simulink model "bubblechase"  (R2015a)
settings: Solver=ode4  SolverMode=MultiTasking  StartTime=0.0  StopTime=inf  FixedStep=BKIN_STEP_TIME  RelTol=1e-3
StartFcn:
  |  warndlg('Dexterit-E models cannot run under simulation. Please compile your model and run it from within Dexterit-E.');set_param(bdroot,'SimulationCommand','stop')
model workspace (MAT data in the model file):
  BKIN_STEP_TIME = 0.00025
  col_x = 1
  col_y = 2
  E_TARGET_ON = 3
  LOGICAL_RADIUS = 4
  START_TARGET_COL = 1
  END_TARGET_COL = 2
  DELAY_POSTTRIAL_COL = 6
  E_STAY_CENTER = 2
  VISUAL_RADIUS = 3
  COLOR = 5
  K_SCORETEXT_ROW = 1
  LABEL_HEIGHT = 9
  E_HIT_TARGET = 5
  E_MISS_TARGET = 9
  K_REWARD_VAL = 2
  K_VIS_RAD = 3
  E_REWARD = 6
  WAIT_AT_START_COL = 3
  LABEL = 8
  K_SCORE_TIME = 4
  HAND_VIS_COL = 9
  DO_REWARD_COL = 10
  E_SHOW_SCORE = 17
  DISPLAY_TRIAL_COL = 11
  BKIN_KINEMATIC_FRAME_SIZE = 400
  E_NO_EVENT = 0
  PAUSE_TIME_COL = 4
  MAXREACH_TIME_COL = 5
  TARGET_XVEL_COL = 7
  TARGET_YVEL_COL = 8
  K_POP_TIME = 5
  K_POP_R_EXPAND = 6
  K_POP_FADE = 7
  STROKE_WIDTH = 6
  STROKE_COLOR = 7
  K_MAX_DIST = 8
  E_TARGET_ESCAPE = 11
  E_END_BREAK = 20
  BTN_BREAK = 2
undefined symbols (not defined in the file or in its folder): slselsubs
libraries: Video x4, General x3, slrtlib x3, simulink x2, KINARM_general x1, xpcnilib x1
(part 1 of 2)
CloseFcn:
  | rtwprivate ssgencode ModelCloseRequest b2lab2d
settings Model: ModifiedComment=chris -- Wed Feb 16 09:18:30 2005 -- Version 1.1384  ModifiedHistory=Feb 16/05 - Add error repeat, add offset ramp  ExtModeArmWhenConnect=off  ExtModeLogAll=off  Creator=Chris Grebeldinger  LastModifiedBy=User
settings SolverCC: EnableConcurrentExecution=on  AutoInsertRateTranBlk=on
settings DataIOCC: LimitDataPoints=off  SignalLoggingSaveFormat=ModelDataLogs  SaveOutput=off  SaveTime=off  SignalLoggingName=sigsOut
settings OptimizationCC: BlockReduction=off  BooleanDataType=off  OptimizeBlockIOStorage=off  BufferReuse=off  GlobalBufferReuse=off  ExpressionFolding=off  ExpressionDepthLimit=2147483647  LocalBlockOutputs=off  InitFltsAndDblsToZero=on
settings DebuggingCC: SaveWithParameterizedLinksMsg=none  UnderspecifiedInitializationDetection=Classic  MergeDetectMultiDrivingBlocksExec=none  SignalResolutionControl=TryResolveAllWithWarning  MultiTaskDSMMsg=warning  FcnCallInpInsideContextMsg=UseLocalSettings  StateNameClashWarn=warning  StrictBusMsg=ErrorOnBusTreatedAsVector
settings HardwareCC: ProdIntDivRoundTo=Zero  ProdEndianess=LittleEndian  ProdLongLongMode=on  ProdHWDeviceType=Generic->32-bit x86 compatible  TargetHWDeviceType=32-bit Generic
settings SFSimCC: SimParseCustomCode=off
settings RTWCC: SystemTargetFile=slrt.tlc  TemplateMakefile=slrt_default_tmf  Description=Simulink Real-Time  CustomSourceCode="#include \"stdio.h\""  RTWCompilerOptimization=on
settings CodeAppCC: MaxIdLength=63
settings SimulinkRealTimeCC: TargetFcnLib=ansi_tfl_tmw.mat  GeneratePreprocessorConditionals=Disable all  xPCisDownloadable=off

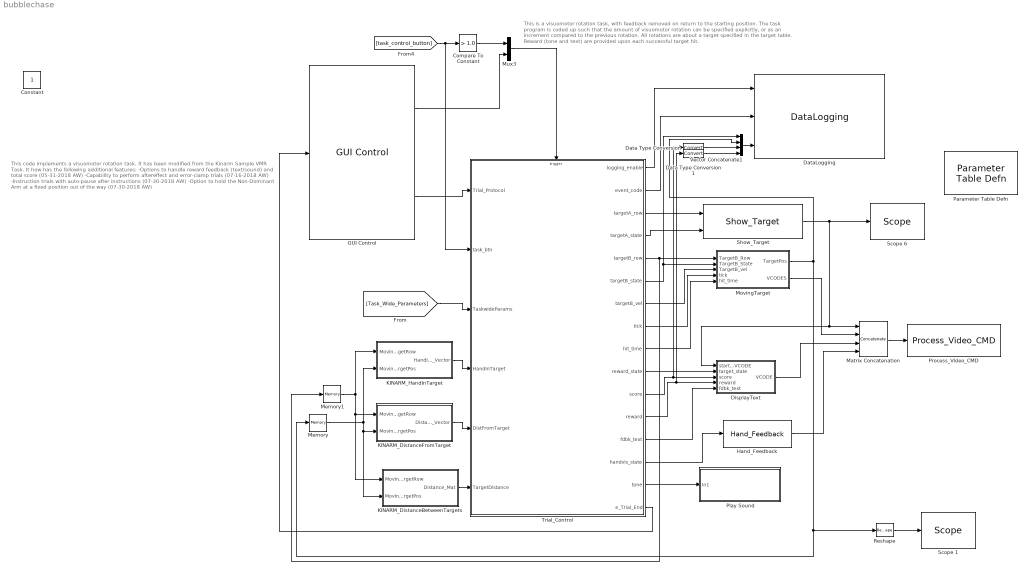
== system bubblechase ==
  note: This code implements a visuomotor rotation task. It has been modified from the Kinarm Sample VMR Task. It how has the following additional features:
      |
      | -Options to handle reward feedback (text/sound) and total score (05-31-2018 AW)
      | -Capability to perform aftereffect and error-clamp trials (07-16-2018 AW)
      | -Instruction trials with auto-pause after instructions (07-30-2018 AW)
      | -Option to hold the Non-Dominant Arm at a fixed position out of the way (07-30-2018 AW)
  note: This is a visuomotor rotation task, with feedback removed on return to the starting position.
      | The task program is coded up such that the amount of visuomotor rotation can be specified explicitly, or as an increment compared to the previous rotation.
      | All rotations are about a target specified in the target table.
      |
      | Reward (tone and text) are provided upon each successful target hit.
  Compare To Constant : simulink/Logic and Bit Operations/Compare To Constant  relop=>  const=1.0  OutDataTypeStr=boolean
  Data Type Conversion : DataTypeConversion
  Data Type Conversion1 : DataTypeConversion
  DataLogging : General/DataLogging  log_event_codes=on  log_analog_inputs=on  show_time_remaining=off  ecat_include=on
  DisplayText : Subsystem
  GUI Control : General/GUI Control  task_version=1.0  show_repeat_trial_flag=off  use_custom_tp=off  target_type_str=Circle  Target_Type=1  XYcols=[1 2]  Vcols=3  Lcols=4  indices_padding=[0 0 0 0;0 0 0 0]  target_table_rows=32  load_table_rows=20  tp_table_rows=50
  Hand_Feedback : KINARM_general/Hand_Feedback  feedback_cntl_src=status only
  KINARM_DistanceBetweenTargets : Subsystem
  KINARM_DistanceFromTarget : Subsystem  mask(KINARM_DistanceFromTarget){use_dominant_hand=on}
      mask prompts: use_dominant_hand "Use "arm to be assessed"?"
      mask help: This block returns a vector corresponding to the Target_Table rows indicating the distance from the specified hand to the center of each of the targets.
      mask init:
      | block_path = gcb;  % store block path, as gcb may change with block operations
      | 
      | %%% Handle background colours if link status changes.  
      | checkBackgroundColour(block_path, 'KINARM_general');
      mask Help:
      | Used to determine the distance from hand (fingertip) to center of targets in the Target_Table.
      | <P>
      | <H2>Library </H2>
      | KINARM general
      | 
      | <H2>Description </H2>
      | This block returns a vector corresponding to the Target_Table rows indicating the distance from the specified hand (fingertip) to the center of each of the targets.
      | <P>
      | The output vector is typically used by a Stateflow chart to affect behavior of the system.  Because this block returns distance-from-target information for all targets in the Target Table, multiple targets can be monitored at once (i.e. the Stateflow chart could have certain transitions that occur if the hand is a given distance from one target versus the distance from a separate target).
      | <P>
      | Because the KINARM_DistanceFromTarget block returns information for only one hand, two copies of this block are required if information for both hands is desired.
      | 
      | <H2>Parameters and Dialog Box</H2>
      | <B>Use "arm to be assessed"?:</B> this checkbox determines which hand is used by this block. In Dexterit-E the operator selects the "arm to be assessed" using radio buttons.
      | When this box is checked the output of this block is derived from the hand information corresponding to the arm selection made by the operator in Dexterit-E.
      | When this box is unchecked the output of this block is derived from the contralateral arm.
      | (Note: to obtain information about both hands, then 2 separate copies of this block are required - one for each hand.)
      | <H2>Related Blocks </H2>
      | DataLogging<BR>
      | KINARM_HandInTarget
  KINARM_HandInTarget : Subsystem  mask(KINARM_HandInTarget){use_dominant_hand=on, target_type=Circle, num_states=1, attribcol1=[LOGICAL_RADIUS], attribcol2=[3], attribcol3=[3], attribcol4=[3], attribcol5=[0]}
      mask prompts: use_dominant_hand "Use "arm to be assessed"?"; target_type "Type of Target"; num_states "Number of Target States"; attribcol1 "State 1 Target Table Column(s)"; attribcol2 "State 2 Target Table Column(s)"; attribcol3 "State 3 Target Table Column(s)"; attribcol4 "State 4 Target Table Column(s)"; attribcol5 "State 5 Target Table Column(s)"
      mask help: This block returns a vector or array corresponding to the Target_Table rows indicating whether the specified hand is in (=1) or out (=0) of each of the targets.
      mask init:
      | block_path = gcb;  % store block path, as gcb may change with block operations
      | 
      | %%% Get the model's workspace, because it is required to evaluate constants from the Parameter Table Def'n block
      | modelName=bdroot(block_path);
      | modelWorkspace = get_param(modelName, 'ModelWorkspace');
      | 
      | %%% Handle background colours if link status changes.  
      | checkBackgroundColour(block_path, 'KINARM_general');
      | 
      | %%% create the names of the input and output ports to display on the mask
      | % Select only the desired states for output. The output port is also renamed to reflect 
      | % whether the output is a vector (in the case of a single state) or an array (of vectors, 
      | % one for each of multiple states).
      | 
      | numStates = str2double( get_param(block_path, 'num_states') );
      | 
      | if numStates == 1
      | 	set_param([block_path '/Selected States'], 'Value', '[1]');
      | 	outputname = 'HandInTarget_Vector';
      | elseif numStates == 2
      | 	set_param([block_path '/Selected States'], 'Value', '[1,2]');
      | 	outputname = 'HandInTarget_Array';
      | elseif numStates == 3
      | 	set_param([block_path '/Selected States'], 'Value', '[1,2,3]');
      | 	outputname = 'HandInTarget_Array';
      | elseif numStates == 4
      | 	set_param([block_path '/Selected States'], 'Value', '[1,2,3,4]');
      | 	outputname = 'HandInTarget_Array';
      | else
      | 	set_param([block_path '/Selected States'], 'Value', '[1,2,3,4,5]');
      | 	outputname = 'HandInTarget_Array';
      | end
      | output_block=char(find_system(gcb,'LookUnderMasks','all','FollowLinks','on','SearchDepth',1,'BlockType','Outport'));
      | set_param(output_block, 'Name', outputname);
      | 
      | 
      | %%%%%%%%%%%%%%%%%%%%%%%%%%%%%%%%%%%%%%%%%%%%%%%%%%%%%%%%%%%%%
      | %%% Check and format the input strings for the vectors of column entires
      | targetTypeStr=get_param(block_path, 'target_type');
      | 
      | switch targetTypeStr(1:3)
      | 	case 'Cir',		numCol = 1;
      | 	case 'Ell',		numCol = 3;
      |     case 'Rec',		numCol = 3;
      |     case 'Lin',		numCol = 3;
      |     case 'Tri',		numCol = 4;
      | 	otherwise,		numCol = 1;
      | end
      | 
      | for ii = 1:5
      | 	variableName = ['attribcol' num2str(ii)];
      | 	attribcoltext = get_param(block_path, variableName);
      | 	attribcoltext = checkUserInputVectorLength(attribcoltext, numCol);
      | 	set_param(block_path, variableName, attribcoltext);
      | end
      | 
      | 
      | %%%%%%%%%%%%%%%%%%%%%%%%%%%%%%%%%%%%%%%%%%%%%%%%%%%%%%%%%%%%%
      | %%% Create the text to show on the mask
      | numStates = str2num(get_param(block_path, 'num_states'));
      | columntext='(columns: ';
      | 
      | for ii = 1:numStates
      | 	variableName = ['attribcol' num2str(ii)];
      | 	attribcolString = get_param(block_path, variableName);
      | 	if isempty(modelWorkspace)
      | 		% if the block is part of a library, then modelWorkspace will be empty and the other code to evaluate attribcolStringEval will fail
      | 		attribcolStringEval = '3';
      | 	else
      | 		[attribcolValue, errorMessage] = BKINevalin(modelWorkspace, attribcolString);
      | 		attribcolStringEval = mat2str( attribcolValue );
      | 	end
      | 	if ii > 1
      | 		columntext = [columntext, '; ', attribcolStringEval];
      | 	else
      | 		columntext = [columntext, attribcolStringEval];
      | 	end
      | end
      | 
      | % Add formatting spaces so that the mask looks nice
      | columntext=strvcat([columntext ')'],' ', ' ');
      mask Help:
      | Used to determine if the hand (fingertip) is in any of the targets in the Target_Table.
      | <P>
      | <B><I>Use of this block requires that the DataLogging block (General library) be set to log KINARM data.</I></B>
      | 
      | <H2>Library </H2>
      | KINARM general
      | 
      | <H2>Description </H2>
      | This block returns a vector or array corresponding to the Target_Table rows indicating whether the specified hand (i.e. fingertip) is in or out of each of the targets.  Each element in the output vector or output array will be either a 0 (hand not in target) or a 1 (hand in target).
      | <P>
      | A vector is returned if only one target state is specified in each target row (see Parameters and Dialog Box), with each index of the vector corresponding to a row in the target table.  An array is returned if more than one target state is specified in a target row, with each row of the array corresponding to a target row and each column corresponding to the nth target state specified in each target row.
      | <P>
      | The output vector or array is typically used by a stateflow chart to affect behavior of the system.  Because this block returns hand-in-target information for all targets in the target table, multiple targets can be monitored at once (i.e. the Stateflow chart could have certain transitions that occur if the hand is in one target and other transitions if it is in a different target).  Likewise, because this block returns hand-in-target information for multiple states of a single target, those multiple states can be monitored simultaneously.
      | <P>
      | Because the KINARM_HandInTarget block returns information for only one hand, two copies of this block are required if information for both hands is desired.
      | <P>
      | 
      | <H2>Parameters and Dialog Box</H2>
      | <B>Use "arm to be assessed"?:</B> this checkbox determines which hand is used by this block. In Dexterit-E the operator selects the "arm to be assessed" using radio buttons.
      | When this box is checked the output of this block is derived from the hand information corresponding to the arm selection made by the operator in Dexterit-E.
      | When this box is unchecked the output of this block is derived from the contralateral arm.
      | (Note: to obtain information about both hands, then 2 separate copies of this block are required - one for each hand.)
      | <P>
      | <B>Type of Target:</B> Enter the type of target specified in the target table:
      | <P>
      | <B>Number of Target States:</B> Enter the number of target states specified in each target row.  Up to four target states are allowed per target row.
      | <P>
      | <B>State <n> Target Table Columns:</B> Enter the columns in the Target Table that specify the relevant target attributes.  Do this for each target state.
      | For a circle, enter the columns corresponding to logical radius (e.g. 4)
      | <BR>For an ellipse, enter the columns corresponding to major radius, minor radius, rotation angle (e.g. [4, 5, 6]).
      | <BR>For a rectangle, enter the columns corresponding to length, height, and rotation angle (e.g. [4, 5, 6]).
      | <BR>For a line, enter the columns corresponding to stroke width, endpoint in x, and endpoint in y (e.g. [3, 4, 5]).
      | <BR>For a triangle, enter the columns corresponding to length, height, peak offset, and rotation angle (e.g. [4, 5, 6, 7]).
      | 
      | <H2>Examples</H2>
      | <B>Example 1.</B>  Suppose a target row will be used to define 1 state for a circle type target and the radius of the visual target is the same radius to be used for determination of hand-in-target.  The related Target Table column is: column 6 = radius.  For this example, "State 1 Target Table Columns" would equal [6].
      | <P>
      | 
      | <B>Example 2.</B>  Suppose a target row will be used to define 1 state for a circle type target, but the radius of the visual target will be different than the radius to be used for determination of hand-in-target.  This option allows independent control over the size of the visual target versus the accuracy needed to be considered "in the target".  The related Target Table columns are: column 6 = radius1 (i.e. radius to target to be drawn); column 7 = radius2 (i.e. radius to be used for hand-in-target) .  For this example, "State 1 Target Table Columns" would equal [7].
      | <P>
      | <B>Example 3.</B>  Suppose a target row will be used to define 2 states for a circle type target, where the radius of the visual target will be a constant, but depending on the state of the system, one of 2 other and different radii will be used for determination of hand-in-target.  The related Target Table columns are: column 6 = radius1 (i.e. radius to target to be drawn); column 7 = radius2 (i.e. radius to be used for hand-in-target for state 1); column 8 = radius3 (i.e. radius to be used for hand-in-target for state 2).  For this example, "State 1 Target Table Columns" would equal [7], while "State 2 Target Table Columns" would equal [8].
      | <P>
      | 
      | <H2>Related Blocks </H2>
      | DataLogging
      mask TypeOptions target_type: Circle | Ellipse | Rectangle | Line | Triangle
      mask Callback target_type:
      | %%%%
      | % Because of bugs iN R2007, R2010a and R2013a (which have been reported to Mathworks), the following code
      | % is required here because in the Initialization Section it will ONLY correctly update those Mask Parameters that are hidden
      | % when the OK button is clicked (NOTE: the initialization code will correctly update all Mask Parameters when the Apply button
      | % is clicked, the bug is that it should also update everything when the OK button is clicked in the absence of an Apply click)
      | %
      | % Adding a set_param call which updates one of the mask parameters will call the initialization code to run, which "avoids"
      | % this bug. This code should be removed once Mathworks has fixed this bug.
      | 
      | temp = get_param(gcb, 'target_type');
      | set_param(gcb, 'target_type', temp);
      mask TypeOptions num_states: 1 | 2 | 3 | 4 | 5
      mask Callback num_states:
      | num_states = str2num(get_param(gcb, 'num_states'));
      | vis = get_param(gcb, 'MaskVisibilities');
      | 
      | % Select only the desired states for output. The output port is also renamed to reflect
      | % whether the output is a vector (in the case of a single state) or an array (of vectors,
      | % one for each of multiple states).
      | output_block=char(find_system(gcb, 'LookUnderMasks', 'all', 'FollowLinks', 'on', 'SearchDepth', 1, 'BlockType', 'Outport'));
      | 
      | if num_states == 1
      | % % % 	set_param([gcb '/Selected States'], 'Value', '[1]');
      | % % % 	set_param(output_block, 'Name', 'HandInTarget_Vector');
      | 	vis{5} = 'off';
      | 	vis{6} = 'off';
      | 	vis{7} = 'off';
      | 	vis{8} = 'off';
      | elseif num_states == 2
      | % % % 	set_param([gcb '/Selected States'], 'Value', '[1,2]');
      | % % % 	set_param(output_block, 'Name', 'HandInTarget_Array');
      | 	vis{5} = 'on';
      | 	vis{6} = 'off';
      | 	vis{7} = 'off';
      | 	vis{8} = 'off';
      | elseif num_states == 3
      | % % % 	set_param([gcb '/Selected States'], 'Value', '[1,2,3]');
      | % % % 	set_param(output_block, 'Name','HandInTarget_Array');
      | 	vis{5} = 'on';
      | 	vis{6} = 'on';
      | 	vis{7} = 'off';
      | 	vis{8} = 'off';
      | elseif num_states == 4
      | % % % 	set_param([gcb '/Selected States'], 'Value', '[1,2,3,4]');
      | % % % 	set_param(output_block, 'Name','HandInTarget_Array');
      | 	vis{5} = 'on';
      | 	vis{6} = 'on';
      | 	vis{7} = 'on';
      | 	vis{8} = 'off';
      | else
      | % % % 	set_param([gcb '/Selected States'], 'Value', '[1,2,3,4,5]');
      | % % % 	set_param(output_block, 'Name', 'HandInTarget_Array');
      | 	vis{5} = 'on';
      | 	vis{6} = 'on';
      | 	vis{7} = 'on';
      | 	vis{8} = 'on';
      | end
      | set_param(gcb, 'MaskVisibilities', vis);
      mask Display:
      | disp(columntext);
      | port_label('output',1,outputname);
  Matrix Concatenation : Concatenate  NumInputs=4  Mode=Multidimensional array
  Memory : Memory  InheritSampleTime=on
  Memory1 : Memory  InheritSampleTime=on
  MovingTarget : Subsystem
  Mux3 : Mux  Inputs=2
  Parameter Table Defn : General/Parameter Table Defn  ShowInLibBrowser=0
  Play Sound : Subsystem
  Process_Video_CMD : Video/Process_Video_CMD  video_delay=50
  Reshape : Reshape
  Scope 1 : slrtlib/Displays and Logging/Scope   scopeno=6  scopetype=Target  autostart=on  viewmode=Numerical  formatstr='%15.6f'  grid=on  ylimits=[0,0]  nosamples=250  noprepostsamples=0  interleave=1  triggermode=FreeRun  triggersignal=1  trigsignalfromport=off  triggerlevel=0.0  triggerslope=Either  triggerscope=1  triggersample=0  filename=data.dat  mode=Lazy  writesize=512  autorestart=off  dynamicfilemode=off  maxwritefilesize=512*1024^2
  Scope 6 : slrtlib/Displays and Logging/Scope   scopeno=4  scopetype=Target  autostart=on  viewmode=Numerical  formatstr='%15.6f'  grid=on  ylimits=[0,0]  nosamples=250  noprepostsamples=0  interleave=1  triggermode=FreeRun  triggersignal=1  trigsignalfromport=off  triggerlevel=0.0  triggerslope=Either  triggerscope=1  triggersample=0  filename=data.dat  mode=Lazy  writesize=512  autorestart=off  dynamicfilemode=off  maxwritefilesize=512*1024^2
  Show_Target : Video/Show_Target  target_type=Circle  num_states=1  attribcol1=[COLOR 0 0 VISUAL_RADIUS]  attribcol2=[0 0 0 0]  attribcol3=[0 0 0 0]  attribcol4=[0 0 0 0]  attribcol5=[0 0 0 0]  stateindices_padding=[0 0 0 0 0 0 0;0 0 0 0 0 0 0;0 0 0 0 0 0 0;0 0 0 0 0 0 0;0 0 0 0 0 0 0]  source=dialog  opacity=100  target_display=Both subject and operator displays  num_col=4
  Trial_Control : Stateflow chart  TreatAsAtomicUnit=on
  Vector Concatenate1 : Concatenate  NumInputs=4
  Constant : Constant  IOType=siggen
  wires:
  Show_Target/1 -> Scope 6/1, DisplayText/1(start_tgt_VCODE), Matrix Concatenation/1
  GUI Control/2 -> Trial_Control/1(Trial_Protocol)
  Trial_Control/16(e_Trial_End) -> GUI Control/1
  Trial_Control/4(targetA_state) -> Show_Target/2
  Trial_Control/3(targetA_row) -> Show_Target/1
  Trial_Control/6(targetB_state) -> MovingTarget/2(TargetB_State), Vector Concatenate1/1
  Trial_Control/2(event_code) -> DataLogging/2
  Matrix Concatenation/1 -> Process_Video_CMD/1
  Hand_Feedback/1 -> Matrix Concatenation/4
  MovingTarget/1(TargetPos) -> Memory/1, Reshape/1, Vector Concatenate1/2
  Trial_Control/1(logging_enable) -> DataLogging/1
  Trial_Control/10(reward_state) -> DisplayText/2(target_state)
  Trial_Control/11(score) -> DisplayText/3(score), Data Type Conversion/1
  [Task_Wide_Parameters] -> Trial_Control/3(TaskwideParams)
  Trial_Control/12(reward) -> Data Type Conversion1/1, DisplayText/4(reward)
  Reshape/1 -> Scope 1/1
  Memory/1 -> KINARM_DistanceFromTarget/2(MovingTargetPos), KINARM_DistanceBetweenTargets/2(MovingTargetPos), KINARM_HandInTarget/2(MovingTargetPos)
  Trial_Control/13(fdbk_text) -> DisplayText/5(fdbk_text)
  DisplayText/1(VCODE) -> Matrix Concatenation/3
  GUI Control/1 -> Mux3/2
  Vector Concatenate1/1 -> DataLogging/3
  Trial_Control/5(targetB_row) -> Memory1/1, MovingTarget/1(TargetB_Row)
  Trial_Control/7(targetB_vel) -> MovingTarget/3(TargetB_vel)
  Trial_Control/8(tick) -> MovingTarget/4(tick)
  MovingTarget/2(VCODES) -> Matrix Concatenation/2
  Trial_Control/14(handvis_state) -> Hand_Feedback/1
  KINARM_HandInTarget/1(HandInTarget_Vector) -> Trial_Control/4(HandInTarget)
  Memory1/1 -> KINARM_HandInTarget/1(MovingTargetRow), KINARM_DistanceBetweenTargets/1(MovingTargetRow), KINARM_DistanceFromTarget/1(MovingTargetRow)
  KINARM_DistanceFromTarget/1(Distance_Vector) -> Trial_Control/5(DistFromTarget)
  KINARM_DistanceBetweenTargets/1(Distance_Mat) -> Trial_Control/6(TargetDistance)
  Trial_Control/9(hit_time) -> MovingTarget/5(hit_time)
  Trial_Control/15(tone) -> Play Sound/1(In1)
  Data Type Conversion/1 -> Vector Concatenate1/3
  Data Type Conversion1/1 -> Vector Concatenate1/4
  [task_control_button] -> Trial_Control/2(task_btn), Compare To Constant/1
  Mux3/1 -> Trial_Control/Trigger
  Compare To Constant/1 -> Mux3/1

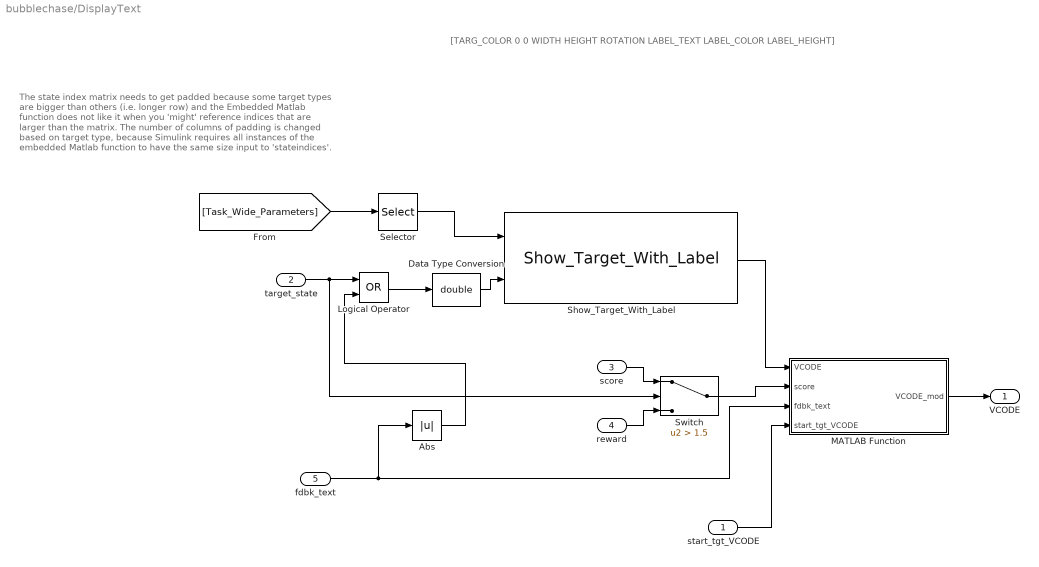
== system bubblechase/DisplayText ==
  note: [TARG_COLOR 0 0 WIDTH HEIGHT ROTATION LABEL_TEXT LABEL_COLOR LABEL_HEIGHT]
  note: The state index matrix needs to get padded because
      | some target types are bigger than others (i.e. longer row)
      | and the Embedded Matlab function does not like it when you
      |  'might' reference indices that are larger than the matrix.
      |
      | The number of columns of padding is changed based on target
      | type, because Simulink requires all instances of the embedded
      | Matlab function to have the same size input to 'stateindices'.
  start_tgt_VCODE : Inport  OutDataTypeStr=double
  target_state : Inport  Port=2  OutDataTypeStr=double
  score : Inport  Port=3  OutDataTypeStr=int32
  reward : Inport  Port=4  OutDataTypeStr=int32
  fdbk_text : Inport  Port=5  OutDataTypeStr=int32
  Abs : Abs
  Data Type Conversion : DataTypeConversion  OutDataTypeStr=double
  Logical Operator : Logic  Operator=OR  AllPortsSameDT=off  OutDataTypeStr=boolean
  MATLAB Function : MATLAB Function  TreatAsAtomicUnit=on
  Selector : Selector  Indices=[K_SCORETEXT_ROW]
  Show_Target_With_Label : Video/Show_Target_With_Label  target_type=Rectangle  num_states=1  attribcol1=[COLOR 0 0 VISUAL_RADIUS VISUAL_RADIUS 0 LABEL COLOR LABEL_HEIGHT]  attribcol2=[0 0 0 0 0 0 0 0 0]  attribcol3=[0 0 0 0 0 0 0 0 0]  attribcol4=[0 0 0 0 0 0 0 0 0]  attribcol5=[0 0 0 0 0 0 0 0 0]  stateindices_padding=[0 0;0 0;0 0;0 0;0 0]  source=dialog  opacity=100  target_display=Both subject and operator displays
  Switch : Switch  Criteria=u2 > Threshold  Threshold=1.5
  VCODE : Outport
  wires:
  target_state/1 -> Logical Operator/1, Switch/2
  Show_Target_With_Label/1 -> MATLAB Function/1(VCODE)
  MATLAB Function/1(VCODE_mod) -> VCODE/1
  score/1 -> Switch/1
  reward/1 -> Switch/3
  Switch/1 -> MATLAB Function/2(score)
  [Task_Wide_Parameters] -> Selector/1
  Selector/1 -> Show_Target_With_Label/1
  fdbk_text/1 -> Abs/1, MATLAB Function/3(fdbk_text)
  Abs/1 -> Logical Operator/2
  Logical Operator/1 -> Data Type Conversion/1
  Data Type Conversion/1 -> Show_Target_With_Label/2
  start_tgt_VCODE/1 -> MATLAB Function/4(start_tgt_VCODE)

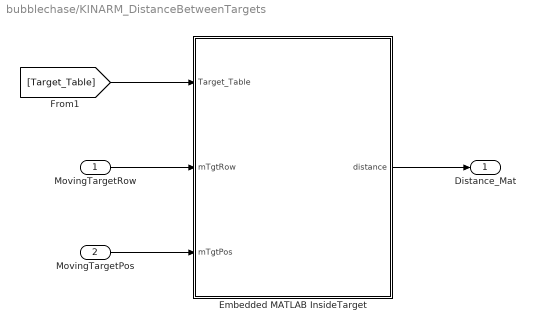
== system bubblechase/KINARM_DistanceBetweenTargets ==
  MovingTargetRow : Inport
  MovingTargetPos : Inport  Port=2
  Embedded MATLAB InsideTarget : MATLAB Function  TreatAsAtomicUnit=on
  Distance_Mat : Outport
  wires:
  Embedded MATLAB InsideTarget/1(distance) -> Distance_Mat/1
  [Target_Table] -> Embedded MATLAB InsideTarget/1(Target_Table)
  MovingTargetRow/1 -> Embedded MATLAB InsideTarget/2(mTgtRow)
  MovingTargetPos/1 -> Embedded MATLAB InsideTarget/3(mTgtPos)

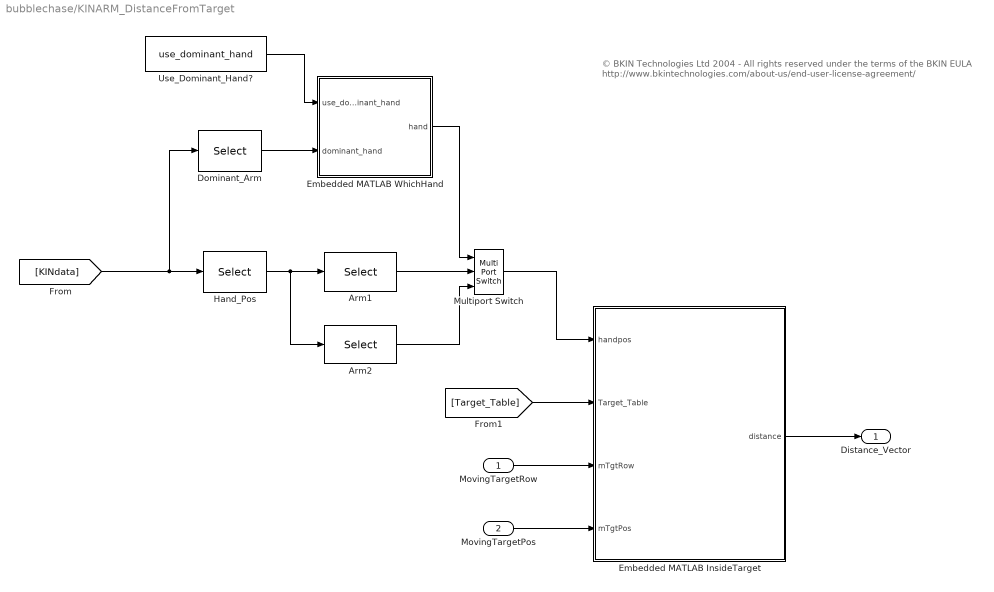
== system bubblechase/KINARM_DistanceFromTarget ==
  note: © BKIN Technologies Ltd 2004  - All rights reserved under the terms of the BKIN EULA
      | http://www.bkintechnologies.com/about-us/end-user-license-agreement/
  MovingTargetRow : Inport
  MovingTargetPos : Inport  Port=2
  Arm1 : Selector  NumberOfDimensions=2  InputPortWidth=3  IndexOptions=Index vector (dialog),Select all  Indices=1,-1  OutputSizes=slselsubs([(-2),(-2)],1),slselsubs([(-2),(-2)],2)
  Arm2 : Selector  NumberOfDimensions=2  InputPortWidth=3  IndexOptions=Index vector (dialog),Select all  Indices=2,-1  OutputSizes=slselsubs([(-2),(-2)],1),slselsubs([(-2),(-2)],2)
  Dominant_Arm : Selector  NumberOfDimensions=2  InputPortWidth=3  IndexOptions=Index vector (dialog),Index vector (dialog)  Indices=[3],[1]  OutputSizes=slselsubs([(-2),(-2)],1),slselsubs([(-2),(-2)],2)
  Embedded MATLAB InsideTarget : MATLAB Function  TreatAsAtomicUnit=on
  Embedded MATLAB WhichHand : MATLAB Function  TreatAsAtomicUnit=on
  Hand_Pos : Selector  NumberOfDimensions=2  InputPortWidth=3  IndexOptions=Select all,Index vector (dialog)  Indices=-1,[23,24]  OutputSizes=slselsubs([(-2),(-2)],1),slselsubs([(-2),(-2)],2)
  Multiport Switch : MultiPortSwitch  Inputs=2
  Use_Dominant_Hand? : Constant  Value=use_dominant_hand
  Distance_Vector : Outport
  wires:
  Embedded MATLAB InsideTarget/1(distance) -> Distance_Vector/1
  Use_Dominant_Hand?/1 -> Embedded MATLAB WhichHand/1(use_dominant_hand)
  Embedded MATLAB WhichHand/1(hand) -> Multiport Switch/1
  [Target_Table] -> Embedded MATLAB InsideTarget/2(Target_Table)
  Multiport Switch/1 -> Embedded MATLAB InsideTarget/1(handpos)
  Arm2/1 -> Multiport Switch/3
  Arm1/1 -> Multiport Switch/2
  Dominant_Arm/1 -> Embedded MATLAB WhichHand/2(dominant_hand)
  Hand_Pos/1 -> Arm2/1, Arm1/1
  [KINdata] -> Dominant_Arm/1, Hand_Pos/1
  MovingTargetRow/1 -> Embedded MATLAB InsideTarget/3(mTgtRow)
  MovingTargetPos/1 -> Embedded MATLAB InsideTarget/4(mTgtPos)

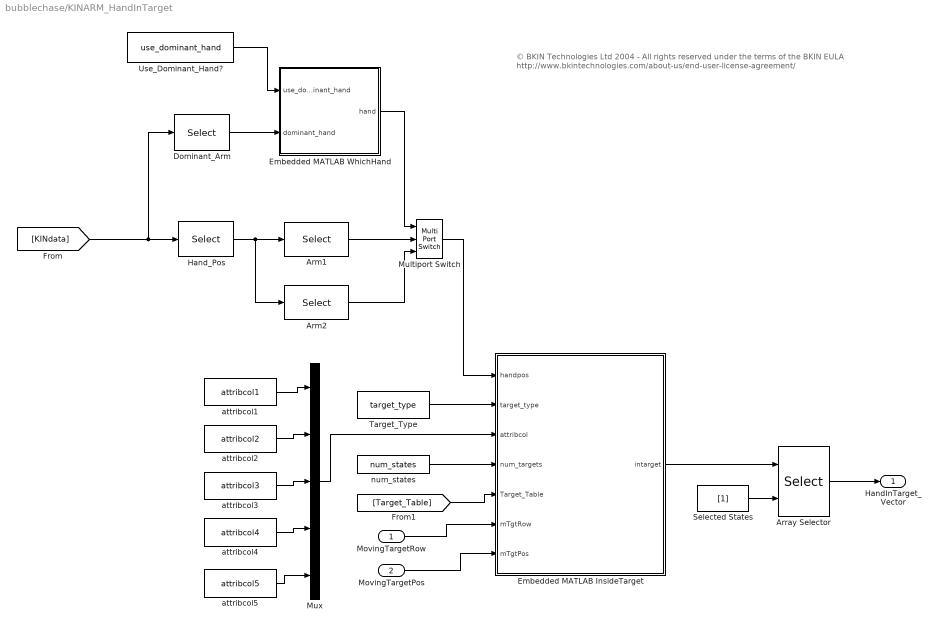
== system bubblechase/KINARM_HandInTarget ==
  note: © BKIN Technologies Ltd 2004  - All rights reserved under the terms of the BKIN EULA
      | http://www.bkintechnologies.com/about-us/end-user-license-agreement/
  MovingTargetRow : Inport
  MovingTargetPos : Inport  Port=2
  Arm1 : Selector  NumberOfDimensions=2  InputPortWidth=3  IndexOptions=Index vector (dialog),Select all  Indices=1,-1  OutputSizes=slselsubs([(-2),(-2)],1),slselsubs([(-2),(-2)],2)
  Arm2 : Selector  NumberOfDimensions=2  InputPortWidth=3  IndexOptions=Index vector (dialog),Select all  Indices=2,-1  OutputSizes=slselsubs([(-2),(-2)],1),slselsubs([(-2),(-2)],2)
  Array Selector : Selector  NumberOfDimensions=2  InputPortWidth=3  IndexOptions=Select all,Index vector (port)  Indices=-1,1  OutputSizes=slselsubs([(-2),(-2)],1),slselsubs([(-2),(-2)],2)
  Dominant_Arm : Selector  NumberOfDimensions=2  InputPortWidth=3  IndexOptions=Index vector (dialog),Index vector (dialog)  Indices=[3],[1]  OutputSizes=slselsubs([(-2),(-2)],1),slselsubs([(-2),(-2)],2)
  Embedded MATLAB InsideTarget : MATLAB Function  TreatAsAtomicUnit=on
      settings: RTWSystemCode=Nonreusable function  RTWFileNameOpts=Use function name
  Embedded MATLAB WhichHand : MATLAB Function  TreatAsAtomicUnit=on
  Hand_Pos : Selector  NumberOfDimensions=2  InputPortWidth=3  IndexOptions=Select all,Index vector (dialog)  Indices=-1,[23,24]  OutputSizes=slselsubs([(-2),(-2)],1),slselsubs([(-2),(-2)],2)
  Multiport Switch : MultiPortSwitch  Inputs=2
  Mux : Mux  Inputs=5
  Selected States : Constant  Value=[1]
  Target_Type : Constant  Value=target_type
  Use_Dominant_Hand? : Constant  Value=use_dominant_hand
  attribcol1 : Constant  Value=attribcol1
  attribcol2 : Constant  Value=attribcol2
  attribcol3 : Constant  Value=attribcol3
  attribcol4 : Constant  Value=attribcol4
  attribcol5 : Constant  Value=attribcol5
  num_states : Constant  Value=num_states
  HandInTarget_Vector : Outport
  wires:
  Selected States/1 -> Array Selector/2
  num_states/1 -> Embedded MATLAB InsideTarget/4(num_targets)
  Mux/1 -> Embedded MATLAB InsideTarget/3(attribcol)
  attribcol4/1 -> Mux/4
  attribcol3/1 -> Mux/3
  attribcol2/1 -> Mux/2
  attribcol1/1 -> Mux/1
  Use_Dominant_Hand?/1 -> Embedded MATLAB WhichHand/1(use_dominant_hand)
  Embedded MATLAB WhichHand/1(hand) -> Multiport Switch/1
  Target_Type/1 -> Embedded MATLAB InsideTarget/2(target_type)
  Array Selector/1 -> HandInTarget_Vector/1
  [Target_Table] -> Embedded MATLAB InsideTarget/5(Target_Table)
  Embedded MATLAB InsideTarget/1(intarget) -> Array Selector/1
  Multiport Switch/1 -> Embedded MATLAB InsideTarget/1(handpos)
  Arm2/1 -> Multiport Switch/3
  Arm1/1 -> Multiport Switch/2
  Dominant_Arm/1 -> Embedded MATLAB WhichHand/2(dominant_hand)
  Hand_Pos/1 -> Arm2/1, Arm1/1
  [KINdata] -> Dominant_Arm/1, Hand_Pos/1
  attribcol5/1 -> Mux/5
  MovingTargetRow/1 -> Embedded MATLAB InsideTarget/6(mTgtRow)
  MovingTargetPos/1 -> Embedded MATLAB InsideTarget/7(mTgtPos)

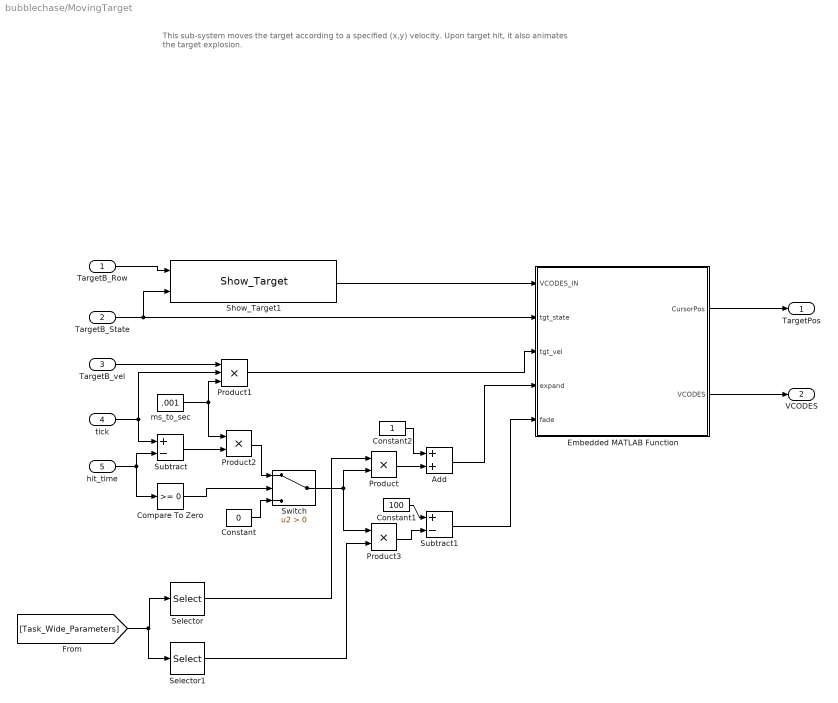
== system bubblechase/MovingTarget ==
  note: This sub-system moves the target according to a specified (x,y) velocity. Upon target hit, it also animates the target explosion.
  TargetB_Row : Inport
  TargetB_State : Inport  Port=2
  TargetB_vel : Inport  Port=3
  tick : Inport  Port=4
  hit_time : Inport  Port=5
  Add : Sum
  Compare To Zero : simulink/Logic and Bit Operations/Compare To Zero  relop=>=  OutDataTypeStr=boolean
  Constant : Constant  Value=0
  Constant1 : Constant  Value=100
  Constant2 : Constant
  Embedded MATLAB Function : MATLAB Function  TreatAsAtomicUnit=on
  Product : Product
  Product1 : Product  Inputs=3
  Product2 : Product
  Product3 : Product
  Selector : Selector  InputPortWidth=50  Indices=[K_POP_R_EXPAND]
  Selector1 : Selector  InputPortWidth=50  Indices=[K_POP_FADE]
  Show_Target1 : Video/Show_Target  target_type=Circle  num_states=2  attribcol1=[COLOR STROKE_COLOR STROKE_WIDTH VISUAL_RADIUS]  attribcol2=[0 STROKE_COLOR STROKE_WIDTH VISUAL_RADIUS]  attribcol3=[0 0 0 0]  attribcol4=[0 0 0 0]  attribcol5=[0 0 0 0]  stateindices_padding=[0 0 0 0 0 0 0;0 0 0 0 0 0 0;0 0 0 0 0 0 0;0 0 0 0 0 0 0;0 0 0 0 0 0 0]  source=dialog  opacity=100  target_display=Both subject and operator displays  num_col=4
  Subtract : Sum  Inputs=+-
  Subtract1 : Sum  Inputs=+-
  Switch : Switch  Criteria=u2 > Threshold
  ms_to_sec : Constant  Value=.001
  TargetPos : Outport
  VCODES : Outport  Port=2
  wires:
  Embedded MATLAB Function/2(VCODES) -> VCODES/1
  Embedded MATLAB Function/1(CursorPos) -> TargetPos/1
  TargetB_Row/1 -> Show_Target1/1
  TargetB_State/1 -> Embedded MATLAB Function/2(tgt_state), Show_Target1/2
  hit_time/1 -> Compare To Zero/1, Subtract/2
  Compare To Zero/1 -> Switch/2
  tick/1 -> Subtract/1, Product1/2
  Switch/1 -> Product/2, Product3/1
  Constant/1 -> Switch/3
  Selector/1 -> Product/1
  Add/1 -> Embedded MATLAB Function/4(expand)
  TargetB_vel/1 -> Product1/1
  Subtract/1 -> Product2/2
  Product2/1 -> Switch/1
  ms_to_sec/1 -> Product2/1, Product1/3
  Product1/1 -> Embedded MATLAB Function/3(tgt_vel)
  Show_Target1/1 -> Embedded MATLAB Function/1(VCODES_IN)
  Product/1 -> Add/2
  Constant2/1 -> Add/1
  Selector1/1 -> Product3/2
  Constant1/1 -> Subtract1/1
  Product3/1 -> Subtract1/2
  Subtract1/1 -> Embedded MATLAB Function/5(fade)
  [Task_Wide_Parameters] -> Selector1/1, Selector/1

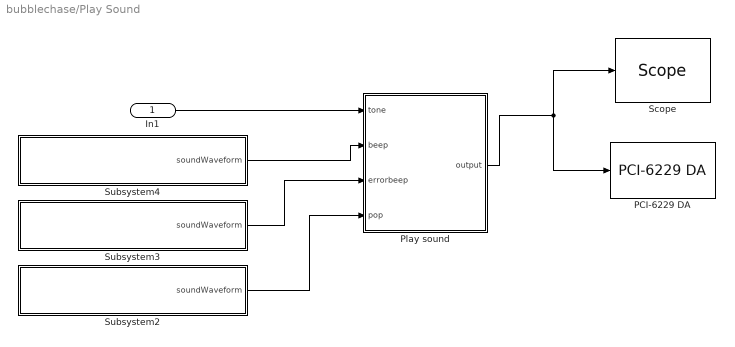
== system bubblechase/Play Sound ==
  In1 : Inport
  PCI-6229 DA : xpcnilib/D//A/M Series/PCI-6229 DA  channel=[1]  reset=[1]  initValue=[0]  sampletime=-1  slot=-1
  Play sound : MATLAB Function  TreatAsAtomicUnit=on
  "Scope " : slrtlib/Displays and Logging/Scope   scopeno=1  scopetype=Target  autostart=on  viewmode=Graphical redraw  formatstr='%15.6f'  grid=on  ylimits=[0,0]  nosamples=4000  noprepostsamples=0  interleave=1  triggermode=FreeRun  triggersignal=1  trigsignalfromport=off  triggerlevel=0.0  triggerslope=Either  triggerscope=1  triggersample=0  filename=data.dat  mode=Lazy  writesize=512  autorestart=off  dynamicfilemode=off  maxwritefilesize=512*1024^2
  Subsystem2 : Subsystem  mask(Load Waveform Into Variable){fileName=pop}
      mask prompts: fileName "Name of .mat Data File (must be in current directory)"
      mask help: This block will load the .MAT file specified in the dialog, and put the first variable into a GoTo called 'soundWaveform'.
      mask init:
      | filenameFromMask = get_param(gcb, 'fileName');
      | 
      | try 
      | 	dataFromFile = load(filenameFromMask);
      | 	names = fieldnames(dataFromFile);
      | 	soundDataFromFile = dataFromFile.(names{1});
      | 	display(['Sound waveform from file ''' filenameFromMask ''' loaded.']);
      | catch ME
      | 	display(ME.message)
      | end
      mask Help:
      | Enter the name a .MAT file containing a single vector or matrix. The .MAT file must be located in the current directory.
      | 
      | The first variable from the .MAT file will be put into a Goto called 'soundWaveform'.
      mask Display: disp(['Load waveform from ''' filenameFromMask ''''])
  Subsystem3 : Subsystem  mask(Load Waveform Into Variable){fileName=errorbeep}
      mask prompts: fileName "Name of .mat Data File (must be in current directory)"
      mask help: This block will load the .MAT file specified in the dialog, and put the first variable into a GoTo called 'soundWaveform'.
      mask init: same as bubblechase/Play Sound/Subsystem2
      mask Help:
      | Enter the name a .MAT file containing a single vector or matrix. The .MAT file must be located in the current directory.
      | 
      | The first variable from the .MAT file will be put into a Goto called 'soundWaveform'.
      mask Display: disp(['Load waveform from ''' filenameFromMask ''''])
  Subsystem4 : Subsystem  mask(Load Waveform Into Variable){fileName=beep1khz}
      mask prompts: fileName "Name of .mat Data File (must be in current directory)"
      mask help: This block will load the .MAT file specified in the dialog, and put the first variable into a GoTo called 'soundWaveform'.
      mask init: same as bubblechase/Play Sound/Subsystem2
      mask Help:
      | Enter the name a .MAT file containing a single vector or matrix. The .MAT file must be located in the current directory.
      | 
      | The first variable from the .MAT file will be put into a Goto called 'soundWaveform'.
      mask Display: disp(['Load waveform from ''' filenameFromMask ''''])
  wires:
  Play sound/1(output) -> PCI-6229 DA/1, "Scope "/1
  Subsystem3/1(soundWaveform) -> Play sound/3(errorbeep)
  Subsystem4/1(soundWaveform) -> Play sound/2(beep)
  In1/1 -> Play sound/1(tone)
  Subsystem2/1(soundWaveform) -> Play sound/4(pop)

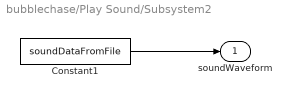
== system bubblechase/Play Sound/Subsystem2 ==
  Constant1 : Constant  Value=soundDataFromFile
  soundWaveform : Outport
  wires:
  Constant1/1 -> soundWaveform/1

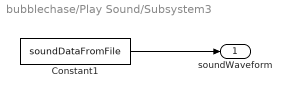
== system bubblechase/Play Sound/Subsystem3 ==
  Constant1 : Constant  Value=soundDataFromFile
  soundWaveform : Outport
  wires:
  Constant1/1 -> soundWaveform/1

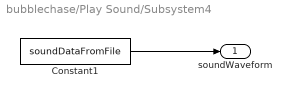
== system bubblechase/Play Sound/Subsystem4 ==
  Constant1 : Constant  Value=soundDataFromFile
  soundWaveform : Outport
  wires:
  Constant1/1 -> soundWaveform/1

== stateflow chart bubblechase/Trial_Control ==
  settings: sampleTime=0.001
  state MainState/
    state StartTargetOn/
      // Turn on first target, wait until hand-is-in-target
      targetA_row = Trial_Protocol[START_TARGET_COL];
      targetA_state=1;
      handvis_state = 1;
      reward_type = Trial_Protocol[DO_REWARD_COL];
      tone = 0;
      reward = TaskwideParams[K_REWARD_VAL];
    state StayAtFirstTarget/
      //log an event, wait for specified period of time.  Hand must STAY in target for specified time.
      event_code=E_STAY_CENTER;
      tickCount =Trial_Protocol[WAIT_AT_START_COL];
    state Show2ndTarget/
      // Turn on second target, log an event, wait for specified delay
      event_code=E_TARGET_ON;
      targetB_row = Trial_Protocol[END_TARGET_COL];
      targetB_vel[1] = 0;
      targetB_vel[2] = 0;
      targetB_state=1;
      tickCount =Trial_Protocol[PAUSE_TIME_COL];
      tick = 0;
      hit_time = -1;
      out_of_bounds1 = 0;
      out_of_bounds2 = 0;
    state Move2ndTarget/
      //Start second target moving
      targetB_state=1;
      targetB_vel[1] = Trial_Protocol[TARGET_XVEL_COL];
      targetB_vel[2] = Trial_Protocol[TARGET_YVEL_COL];
      tickCount =Trial_Protocol[MAXREACH_TIME_COL]-Trial_Protocol[PAUSE_TIME_COL];
      during:
      on e_clk: tick++;
      hit_time = tick;
      out_of_bounds1 = (TargetDistance[targetA_row][targetB_row] > TaskwideParams[K_MAX_DIST]);
      out_of_bounds2 = (TargetDistance[targetA_row][targetB_row] < 0.01);
    state TargetNotCaptured/
      //if target exceeds workspace bounds, trial is over
      event_code = E_TARGET_ESCAPE;
      targetB_vel[1] = 0;
      targetB_vel[2] = 0;
      targetB_state=0;
      reward_state = 1; //allow feedback text
      fdbk_text = -1;
      tickCount = 1000;
    state Miss2ndTarget/
      //if hand exceeds target, trial is over
      event_code = E_MISS_TARGET;
      targetB_vel[1] = 0;
      targetB_vel[2] = 0;
      targetB_state=0;
      reward_state = 0;
      fdbk_text = -1;
      tickCount = 500;
    state Hit2ndTarget/
      // change the 2nd target's state, log an event, wait for the rest of the trial to end
      event_code=E_HIT_TARGET;
    state TooSlowState/
      fdbk_text = -2;  //"too slow"
      reward_state = 1; //allow feedback text
      targetB_vel[1] = 0;
      targetB_vel[2] = 0;
      targetB_state=0;
      tickCount = 1000;
    state DoReward/
      event_code = E_REWARD;
      targetB_state=2;
      reward_state=1;
      reward = TaskwideParams[K_REWARD_VAL];
      score += reward;
      fdbk_text = 1;
      tone = 1;
      tickCount = TaskwideParams[K_POP_TIME];
      during:
      on e_clk: tick++;
    state NoReward/
      targetB_state=0;
      reward_state = 0;
      fdbk_text = 0;
      tone = 0;
      tickCount = TaskwideParams[K_POP_TIME];
      score += 0;
      //do nothing
      during:
      on e_clk: tick++;
    state NoRewardText/
      event_code = E_REWARD;
      targetB_state=2;
      reward_state = 0;
      fdbk_text = 0;
      tone = 1;
      tickCount = TaskwideParams[K_POP_TIME];
      score += 0;
      //do nothing
      during:
      on e_clk: tick++;
    state EndOfTrial/
      // Shut off the chase target
      targetB_vel[1] = 0;
      targetB_vel[2] = 0;
      targetB_state=0;
    StartTargetOn -> StayAtFirstTarget : [HandInTarget[targetA_row]==1]
    StayAtFirstTarget -> StartTargetOn [order 2] : [HandInTarget[targetA_row]==0]
    StayAtFirstTarget -> Show2ndTarget [order 1] : after(tickCount, e_clk)
    Show2ndTarget -> Move2ndTarget : after(tickCount,e_clk)
    TooSlowState -> Move2ndTarget [order 1] : after(tickCount,e_clk)
        | //time out if movement taking too long
    Move2ndTarget -> TargetNotCaptured [order 1] : [out_of_bounds1 || out_of_bounds2]
    Move2ndTarget -> Hit2ndTarget [order 3] : [HandInTarget[targetB_row]==1]
    Move2ndTarget -> Miss2ndTarget [order 2] : [DistFromTarget[targetA_row] >= TargetDistance[targetA_row][targetB_row]]
    Hit2ndTarget -> DoReward [order 3] : [reward_type == 1]
        | //do the reward and fdbk
    Hit2ndTarget -> NoReward [order 2] : [reward_type == 0]
        | //no reward or feedback
    Hit2ndTarget -> NoRewardText [order 1] : [reward_type == 2]
        | //no reward but fdbk
    TargetNotCaptured -> EndOfTrial : after(tickCount,e_clk)
    Miss2ndTarget -> EndOfTrial : after(tickCount, e_clk)
    TooSlowState -> EndOfTrial [order 2] : after(tickCount, e_clk)
    DoReward -> EndOfTrial : after(tickCount, e_clk)
    NoReward -> EndOfTrial : after(tickCount, e_clk)
    NoRewardText -> EndOfTrial : after(tickCount, e_clk)
  state Initialize/
    // Turn off both targets, set hand_feedback on
    targetA_state=0;
    targetB_state=0;
    reward_state = 0;
    score = 0;
    handvis_state = 1;
    reward_type = 0;
    fdbk_text = 0;
    tone = 0;
    logging_enable = 1;
  state Ending/
    //end the special "show score" state
    e_Trial_End;
    event_code = E_END_BREAK;
    reward_state = 0;
    fdbk_text = 0;
    handvis_state = 1;
    targetA_state = 1;
    tickCount = 800;
  state ReturnToStart1/
    targetA_state=1;
    handvis_state = 1;
    reward_state = 0;
    logging_enable = 1;
  state ShowScoreState/
    event_code = E_SHOW_SCORE;
    targetA_state = 0;
    targetB_state = 0;
    handvis_state = 1;
    reward_state = 2;
    fdbk_text = Trial_Protocol[DISPLAY_TRIAL_COL];
    tickCount = TaskwideParams[K_SCORE_TIME];
    logging_enable = 0;
  state Inter_Trial_State/
    // send e_Trial_End event
    e_Trial_End;
    // turn off both targets
    // stop data logging
    event_code=0;
    targetA_state=1; //don't shut off
    targetB_state=0;
    reward_state = 0;
    fdbk_text = 0;
  state ReturnToStart/
    //targetA_state=1;
    handvis_state = 1;
    reward_state = 0; //shut off feedback
    tickCount =50;
  state Inter_Trial_Hold/
    //temporarily hold here
    tickCount = Trial_Protocol[DELAY_POSTTRIAL_COL];
  (default) -> Initialize
  Initialize -> StartTargetOn : after(1,e_clk)
  ReturnToStart1 -> StartTargetOn : after(1, e_clk)
  Ending -> ReturnToStart1 : after(tickCount,e_clk)/
      | //continue if a regular trial comes after!
  ShowScoreState -> Ending : [after(tickCount,e_clk) && task_btn > 0]
  (junction 74) -> ReturnToStart1 [order 1] : [Trial_Protocol[DISPLAY_TRIAL_COL] == 0]
  (junction 74) -> ShowScoreState [order 2] : [Trial_Protocol[DISPLAY_TRIAL_COL] > 0]
  Inter_Trial_State -> (junction 74) : after(1,e_clk)
  MainState -> Inter_Trial_State : e_ExitTrialNow/
      | // if e_ExitTrialNow event occurs...
      | tickCount=1;
  ReturnToStart -> Inter_Trial_State : after(tickCount,e_clk)
  Inter_Trial_Hold -> ReturnToStart : [ DistFromTarget[targetA_row] <= TaskwideParams[K_VIS_RAD] && after(tickCount,e_clk) ]
      | //if the hand is close to the start, turn vision of the hand back on
  EndOfTrial -> Inter_Trial_Hold
  data: logging_enable output boolean; event_code output double; Trial_Protocol input double; task_btn input double; targetA_row output [1..32]; targetA_state output double; targetB_row output double; targetB_state output double; targetB_vel output double size=[2 1]; tick output int32; hit_time output int32; tickCount local double; reward_state output double; score output int32; reward output int32; fdbk_text output int32; handvis_state output double; TaskwideParams input double; HandInTarget input double; DistFromTarget input double; TargetDistance input double; tone output double; reward_type local double; out_of_bounds1 local boolean =0; out_of_bounds2 local boolean =0
  data targetA_row settings: description=index of the row currently being used in the TargetTable
  events: e_button input EITHER_EDGE_EVENT; e_clk input RISING_EDGE_EVENT; e_ExitTrialNow input EITHER_EDGE_EVENT; e_Trial_End output EITHER_EDGE_EVENT
